simulink model "ctrl_student___for_MCLAB_org"  (Simulink 10.0)
settings: Solver=ode4  StartTime=0.0  StopTime=inf  FixedStep=0.01  RelTol=1e-3  EnableMultiTasking=on
(part 2 of 2)

== matlab function tau to real ship (only use in MCLab)/Limited allocation: VSP only  in surge and BT only in yaw ==
  data: X_VSP input double; u_BT output double; N_BT input double; u_VSP output double; alpha_VSP output double; omega_VSP output double
function [u_BT,u_VSP,alpha_VSP,omega_VSP]= fcn(X_VSP,N_BT)

l_BT     = 0.3875;
F_max_BT = 2.629;
u_BT     = N_BT/(l_BT*F_max_BT);

omega_VSP = 0.3;
F_max_VSP = 1.165;
u_VSP     = abs(X_VSP)/(2*F_max_VSP);
alpha_VSP = pi*(X_VSP<=0); % 0 if positive X_VSP, pi if negative

== matlab function Noise generator/Sample & hold/MATLAB Function1 ==
  data: counter input double; input input double; hold input double; output output double
function output = fcn(counter,input,hold)
%#codegen

if counter == 0
    output = input;
else
    output = hold;
end
